simulink model "net_test"  (R2024a)
settings: Solver=FixedStepDiscrete  StartTime=0.0  StopTime=1000  RelTol=1e-3
values from neighbouring files (symbols this model uses):
  sigma = 0.1    [try_theta.m]
  theta = [-0.675635383614 0.588569081368 -0.37756991591 0.0570662710124 -0.668702541 0.203963882803 -0.47405743092 0.308158196954 0.37842900628 0.496303185647 -0.098916802995 -0.832357244006 ... (20 elements, 1x20)]    [big_net1.mat]    (also in big_net2.mat = [0.502534118611 -0.489809769081 0.0119141033303 0.3981534453; try_theta.m = 2*rand(1,2*M)-1)
settings Model: Creator=jogal  LastModifiedBy=jogal
settings OptimizationCC: ReuseModelBlockBuffer=off
settings RTWCC: GPUComputeCapability=3.5

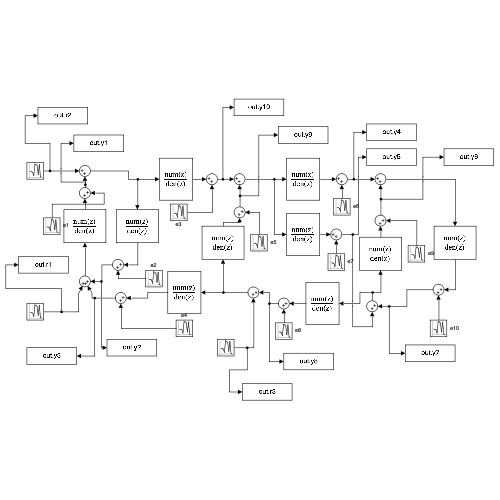
[thumbnail: Simulink's stored preview of the top-level diagram]
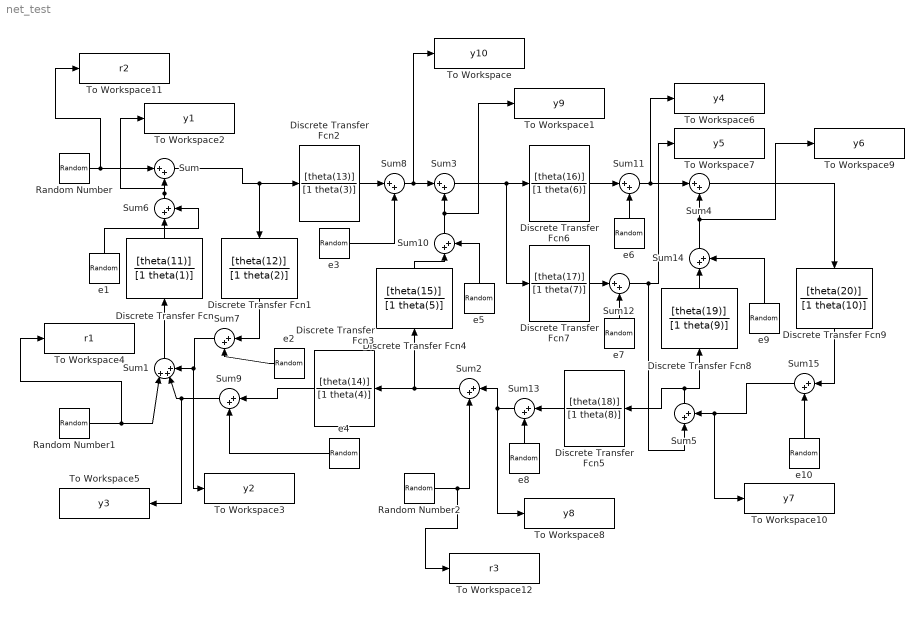
== system net_test ==
  Discrete Transfer Fcn : DiscreteTransferFcn  Numerator=[theta(11)]  Denominator=[1 theta(1)]
  Discrete Transfer Fcn1 : DiscreteTransferFcn  Numerator=[theta(12)]  Denominator=[1 theta(2)]
  Discrete Transfer Fcn2 : DiscreteTransferFcn  Numerator=[theta(13)]  Denominator=[1 theta(3)]
  Discrete Transfer Fcn3 : DiscreteTransferFcn  Numerator=[theta(14)]  Denominator=[1 theta(4)]
  Discrete Transfer Fcn4 : DiscreteTransferFcn  Numerator=[theta(15)]  Denominator=[1 theta(5)]
  Discrete Transfer Fcn5 : DiscreteTransferFcn  Numerator=[theta(18)]  Denominator=[1 theta(8)]
  Discrete Transfer Fcn6 : DiscreteTransferFcn  Numerator=[theta(16)]  Denominator=[1 theta(6)]
  Discrete Transfer Fcn7 : DiscreteTransferFcn  Numerator=[theta(17)]  Denominator=[1 theta(7)]
  Discrete Transfer Fcn8 : DiscreteTransferFcn  Numerator=[theta(19)]  Denominator=[1 theta(9)]
  Discrete Transfer Fcn9 : DiscreteTransferFcn  Numerator=[theta(20)]  Denominator=[1 theta(10)]
  Random Number : RandomNumber  Seed=2  SampleTime=1
  Random Number1 : RandomNumber  Seed=1  SampleTime=1
  Random Number2 : RandomNumber  Seed=3  SampleTime=1
  Sum{,2..15} (15 alike) : Sum  Inputs=|++
  Sum1 : Sum  Inputs=|+++
  To Workspace : ToWorkspace  VariableName=y10  SampleTime=-1
  To Workspace1 : ToWorkspace  VariableName=y9  SampleTime=-1
  To Workspace10 : ToWorkspace  VariableName=y7  SampleTime=-1
  To Workspace11 : ToWorkspace  VariableName=r2  SampleTime=-1
  To Workspace12 : ToWorkspace  VariableName=r3  SampleTime=-1
  To Workspace2 : ToWorkspace  VariableName=y1  SampleTime=-1
  To Workspace3 : ToWorkspace  VariableName=y2  SampleTime=-1
  To Workspace4 : ToWorkspace  VariableName=r1  SampleTime=-1
  To Workspace5 : ToWorkspace  VariableName=y3  SampleTime=-1
  To Workspace6 : ToWorkspace  VariableName=y4  SampleTime=-1
  To Workspace7 : ToWorkspace  VariableName=y5  SampleTime=-1
  To Workspace8 : ToWorkspace  VariableName=y8  SampleTime=-1
  To Workspace9 : ToWorkspace  VariableName=y6  SampleTime=-1
  e{1..10} (10 alike) : RandomNumber  Variance=sigma  SampleTime=1
  wires:
  Sum/1 -> Discrete Transfer Fcn1/1, Discrete Transfer Fcn2/1
  Sum1/1 -> Discrete Transfer Fcn/1
  Sum2/1 -> Discrete Transfer Fcn3/1, Discrete Transfer Fcn4/1
  Sum3/1 -> Discrete Transfer Fcn7/1, Discrete Transfer Fcn6/1
  Sum5/1 -> Discrete Transfer Fcn5/1, Discrete Transfer Fcn8/1
  Sum4/1 -> Discrete Transfer Fcn9/1
  Random Number/1 -> To Workspace11/1, Sum/1
  Random Number1/1 -> To Workspace4/1, Sum1/1
  Random Number2/1 -> To Workspace12/1, Sum2/2
  Sum6/1 -> To Workspace2/1, Sum/2
  Discrete Transfer Fcn/1 -> Sum6/1
  e1/1 -> Sum6/2
  Discrete Transfer Fcn1/1 -> Sum7/1
  Sum7/1 -> To Workspace3/1, Sum1/3
  e2/1 -> Sum7/2
  Discrete Transfer Fcn2/1 -> Sum8/1
  e3/1 -> Sum8/2
  Sum8/1 -> To Workspace/1, Sum3/1
  Discrete Transfer Fcn3/1 -> Sum9/1
  e4/1 -> Sum9/2
  Sum9/1 -> To Workspace5/1, Sum1/2
  Discrete Transfer Fcn4/1 -> Sum10/1
  e5/1 -> Sum10/2
  Discrete Transfer Fcn6/1 -> Sum11/1
  Sum11/1 -> To Workspace6/1, Sum4/1
  e6/1 -> Sum11/2
  Discrete Transfer Fcn7/1 -> Sum12/1
  e7/1 -> Sum12/2
  Sum12/1 -> To Workspace7/1, Sum5/1
  Discrete Transfer Fcn5/1 -> Sum13/1
  Sum13/1 -> Sum2/1, To Workspace8/1
  Sum10/1 -> To Workspace1/1, Sum3/2
  e8/1 -> Sum13/2
  Discrete Transfer Fcn8/1 -> Sum14/1
  Sum14/1 -> To Workspace9/1, Sum4/2
  e9/1 -> Sum14/2
  Discrete Transfer Fcn9/1 -> Sum15/1
  e10/1 -> Sum15/2
  Sum15/1 -> To Workspace10/1, Sum5/2
